simulink model "FaMe_HA1_Model"  (R2014a)
settings: Solver=ode1  StartTime=0.0  StopTime=20.0  FixedStep=0.0001  RelTol=1e-3
values from neighbouring files (symbols this model uses):
  A = 0.3    [FaMe_HA1_i.m]    (also in FaMe_HA1_ii.m)
  alpha = 5    [FaMe_HA1_i.m]    (also in FaMe_HA1_ii.m)
  cw = 0.8    [FaMe_HA1_i.m]    (also in FaMe_HA1_ii.m)
  f = 0.04    [FaMe_HA1_i.m]    (also in FaMe_HA1_ii.m)
  g = 9.81    [FaMe_HA1_i.m]    (also in FaMe_HA1_ii.m)
  J = 0.0015    [FaMe_HA1_i.m]    (also in FaMe_HA1_ii.m)
  kM = 0.1    [FaMe_HA1_i.m]    (also in FaMe_HA1_ii.m)
  kV = 0.0005    [FaMe_HA1_i.m]    (also in FaMe_HA1_ii.m)
  L = 0.001    [FaMe_HA1_i.m]    (also in FaMe_HA1_ii.m)
  m = 20    [FaMe_HA1_i.m]    (also in FaMe_HA1_ii.m)
  R = 5    [FaMe_HA1_i.m]    (also in FaMe_HA1_ii.m)
  r_dyn = 0.06    [FaMe_HA1_i.m]    (also in FaMe_HA1_ii.m)
  rho = 1.2    [FaMe_HA1_i.m]    (also in FaMe_HA1_ii.m)
  t_hold = 0    [FaMe_HA1_i.m]    (also in FaMe_HA1_ii.m = 5)
  Ue = 21.375    [FaMe_HA1_i.m]    (also in FaMe_HA1_ii.m = 12.508)
  v_switch = 0    [FaMe_HA1_i.m]    (also in FaMe_HA1_ii.m = 10)
settings Model: Creator=Tom-Morten  LastModifiedBy=Tom-Morten

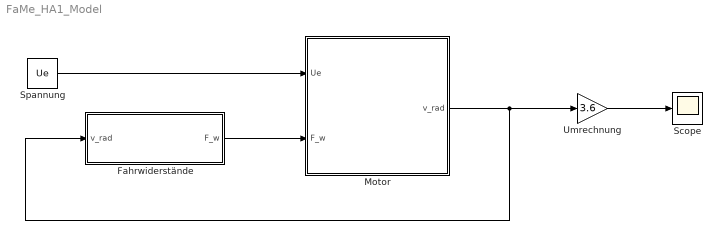
== system FaMe_HA1_Model ==
  Fahrwiderstände : Subsystem
  Motor : Subsystem
  Scope : Scope
      settings: TimeRange=10  YMin=-500  YMax=50  SampleInput=on
  Spannung : Constant  Value=Ue
  Umrechnung : Gain  Gain=3.6
  wires:
  Spannung/1 -> Motor/1(Ue)
  Fahrwiderstände/1(F_w) -> Motor/2(F_w)
  Motor/1(v_rad) -> Umrechnung/1, Fahrwiderstände/1(v_rad)
  Umrechnung/1 -> Scope/1

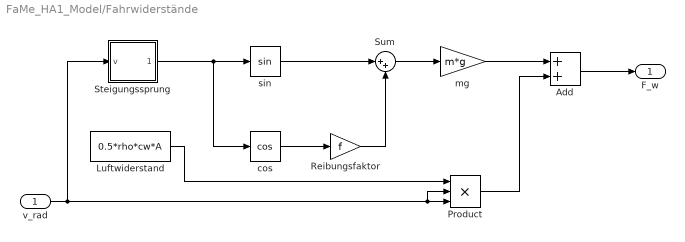
== system FaMe_HA1_Model/Fahrwiderstände ==
  v_rad : Inport
  Add : Sum
  Luftwiderstand : Constant  Value=0.5*rho*cw*A
  Product : Product  Inputs=3
  Reibungsfaktor : Gain  Gain=f
  Steigungssprung : Subsystem
  Sum : Sum  Inputs=|++
  cos : Trigonometry  Operator=cos
  mg : Gain  Gain=m*g
  sin : Trigonometry
  F_w : Outport
  wires:
  Luftwiderstand/1 -> Product/1
  v_rad/1 -> Product/2, Product/3, Steigungssprung/1(v)
  Add/1 -> F_w/1
  Product/1 -> Add/2
  cos/1 -> Reibungsfaktor/1
  Sum/1 -> mg/1
  Reibungsfaktor/1 -> Sum/2
  sin/1 -> Sum/1
  Steigungssprung/1(alpha) -> sin/1, cos/1
  mg/1 -> Add/1

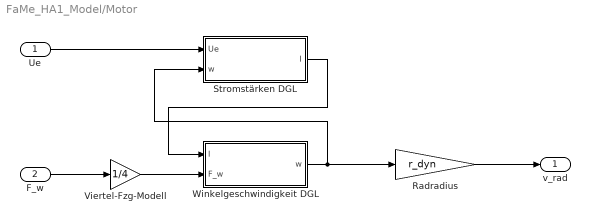
== system FaMe_HA1_Model/Motor ==
  Ue : Inport
  F_w : Inport  Port=2
  Radradius : Gain  Gain=r_dyn
  Stromstärken DGL : Subsystem
  Viertel-Fzg-Modell : Gain  Gain=1/4
  Winkelgeschwindigkeit DGL : Subsystem
  v_rad : Outport
  wires:
  Ue/1 -> Stromstärken DGL/1(Ue)
  F_w/1 -> Viertel-Fzg-Modell/1
  Radradius/1 -> v_rad/1
  Stromstärken DGL/1(I) -> Winkelgeschwindigkeit DGL/1(I)
  Winkelgeschwindigkeit DGL/1(w) -> Radradius/1, Stromstärken DGL/2(w)
  Viertel-Fzg-Modell/1 -> Winkelgeschwindigkeit DGL/2(F_w)

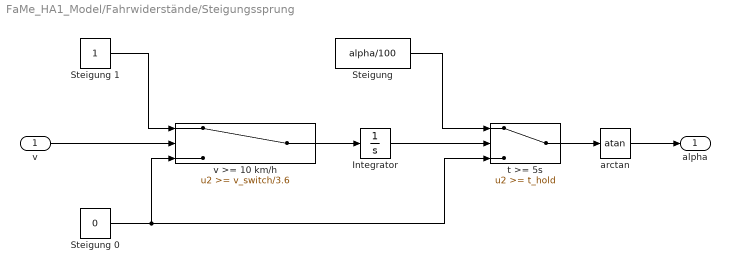
== system FaMe_HA1_Model/Fahrwiderstände/Steigungssprung ==
  v : Inport
  Integrator : Integrator
  Steigung : Constant  Value=alpha/100
  Steigung 0 : Constant  Value=0
  Steigung 1 : Constant
  arctan : Trigonometry  Operator=atan
  t >= 5s : Switch  Threshold=t_hold
  v >= 10 km/h : Switch  Threshold=v_switch/3.6
  alpha : Outport
  wires:
  v/1 -> v >= 10 km/h/2
  arctan/1 -> alpha/1
  Steigung 1/1 -> v >= 10 km/h/1
  v >= 10 km/h/1 -> Integrator/1
  Integrator/1 -> t >= 5s/2
  Steigung/1 -> t >= 5s/1
  Steigung 0/1 -> t >= 5s/3, v >= 10 km/h/3
  t >= 5s/1 -> arctan/1

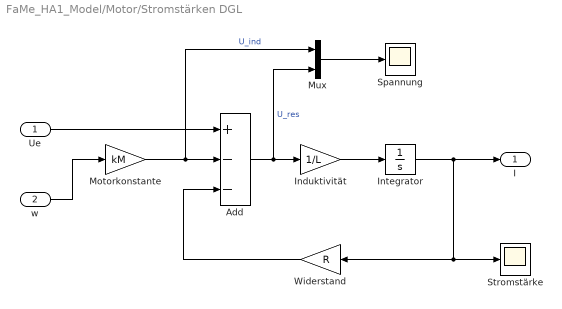
== system FaMe_HA1_Model/Motor/Stromstärken DGL ==
  Ue : Inport
  w : Inport  Port=2
  Add : Sum  Inputs=+--
  Induktivität : Gain  Gain=1/L
  Integrator : Integrator
  Motorkonstante : Gain  Gain=kM
  Mux : Mux  Inputs=2
  Spannung : Scope
      settings: ShowLegends=on
  Stromstärke : Scope
      settings: SaveName=ScopeData2
  Widerstand : Gain  Gain=R
  I : Outport
  wires:
  Ue/1 -> Add/1
  w/1 -> Motorkonstante/1
  Add/1 -> Mux/2, Induktivität/1  "U_res"
  Widerstand/1 -> Add/3
  Motorkonstante/1 -> Mux/1, Add/2  "U_ind"
  Induktivität/1 -> Integrator/1
  Integrator/1 -> I/1, Stromstärke/1, Widerstand/1
  Mux/1 -> Spannung/1

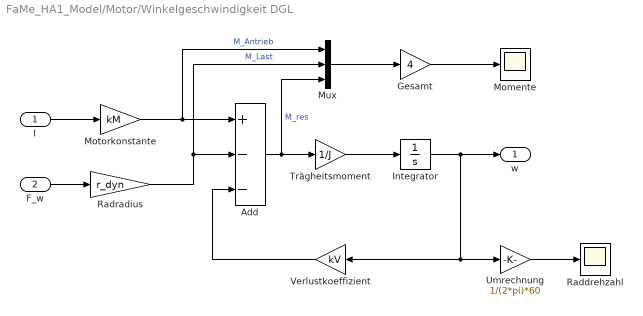
== system FaMe_HA1_Model/Motor/Winkelgeschwindigkeit DGL ==
  I : Inport
  F_w : Inport  Port=2
  Add : Sum  Inputs=+--
  Gesamt : Gain  Gain=4
  Integrator : Integrator
  Momente : Scope
      settings: ShowLegends=on  SaveName=ScopeData3
  Motorkonstante : Gain  Gain=kM
  Mux : Mux  Inputs=3
  Raddrehzahl : Scope
      settings: TimeRange=10  YMin=0  YMax=600  SaveName=ScopeData4
  Radradius : Gain  Gain=r_dyn
  Trägheitsmoment : Gain  Gain=1/J
  Umrechnung : Gain  Gain=1/(2*pi)*60
  Verlustkoeffizient : Gain  Gain=kV
  w : Outport
  wires:
  I/1 -> Motorkonstante/1
  F_w/1 -> Radradius/1
  Motorkonstante/1 -> Mux/1, Add/1  "M_Antrieb"
  Radradius/1 -> Mux/2, Add/2  "M_Last"
  Add/1 -> Mux/3, Trägheitsmoment/1  "M_res"
  Trägheitsmoment/1 -> Integrator/1
  Integrator/1 -> w/1, Umrechnung/1, Verlustkoeffizient/1
  Verlustkoeffizient/1 -> Add/3
  Mux/1 -> Gesamt/1
  Umrechnung/1 -> Raddrehzahl/1
  Gesamt/1 -> Momente/1
